simulink model "MPC_KIN_IPOPT_fast_no_param"  (R2018b)
settings: Solver=ode4  StartTime=0.0  StopTime=inf  FixedStep=Tsample  RelTol=1e-3
values from neighbouring files (symbols this model uses):
  N = evalin('base', 'N')    [solver_NLP_no_param.m]
undefined symbols (not defined in the file or in its folder): DiscIntNeverNeededParam, T, Tsample, x0_val, xd
libraries: simulink x2, templibrary x1
settings Model: Creator=francesco  LastModifiedBy=francesco
settings ModelReferenceCC: PropagateVarSize=Only when enabling

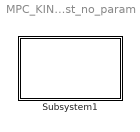
== system MPC_KIN_IPOPT_fast_no_param ==
  Subsystem1 : Subsystem  InitFcn=initialization_no_param

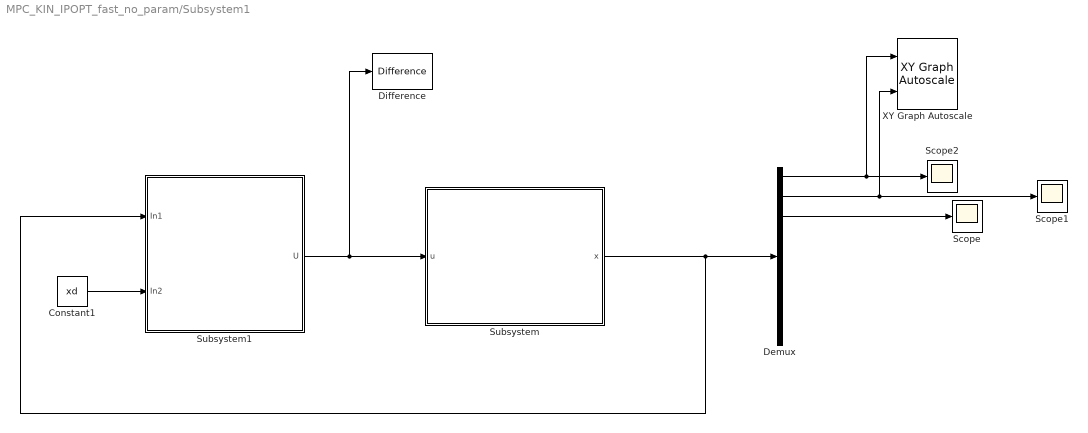
== system MPC_KIN_IPOPT_fast_no_param/Subsystem1 ==
  Constant1 : Constant  Value=xd
  Demux : Demux  Outputs=9
  Difference : simulink/Discrete/Difference  ICPrevInput=0.0  OutMin=[]  OutMax=[]  OutDataType=fixdt(1, 16)  OutScaling=2^-10  DoSatur=off
  Scope : Scope
  Scope1 : Scope
  Scope2 : Scope
  Subsystem : Subsystem
      mask Display: disp('{\bf\fontsize{10}KINEMATIC SYSTEM}', 'texmode','on');
  Subsystem1 : Subsystem
  XY Graph Autoscale : templibrary/XY Graph  Autoscale  xmin=-1  xmax=1  ymin=-1  ymax=1  st=-1
  wires:
  Subsystem/1(x) -> Demux/1, Subsystem1/1(In1)
  Demux/1 -> XY Graph Autoscale/1, Scope2/1
  Demux/3 -> Scope/1
  Demux/2 -> XY Graph Autoscale/2, Scope1/1
  Subsystem1/1(U) -> Difference/1, Subsystem/1(u)
  Constant1/1 -> Subsystem1/2(In2)

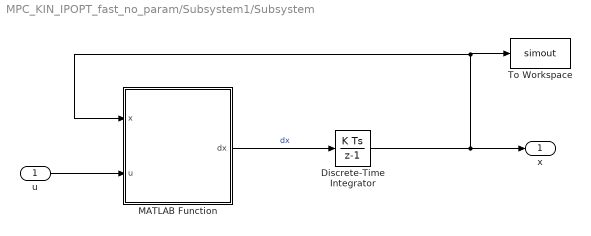
== system MPC_KIN_IPOPT_fast_no_param/Subsystem1/Subsystem ==
  u : Inport
  Discrete-Time Integrator : DiscreteIntegrator  InitialCondition=x0_val  SampleTime=Tsample  ICPrevOutput=DiscIntNeverNeededParam  ICPrevScaledInput=DiscIntNeverNeededParam
  MATLAB Function : MATLAB Function  TreatAsAtomicUnit=on
  To Workspace : ToWorkspace  VariableName=simout  SampleTime=T
  x : Outport  SampleTime=Tsample
  wires:
  u/1 -> MATLAB Function/2(u)
  MATLAB Function/1(dx) -> Discrete-Time Integrator/1  "dx"
  Discrete-Time Integrator/1 -> MATLAB Function/1(x), To Workspace/1, x/1

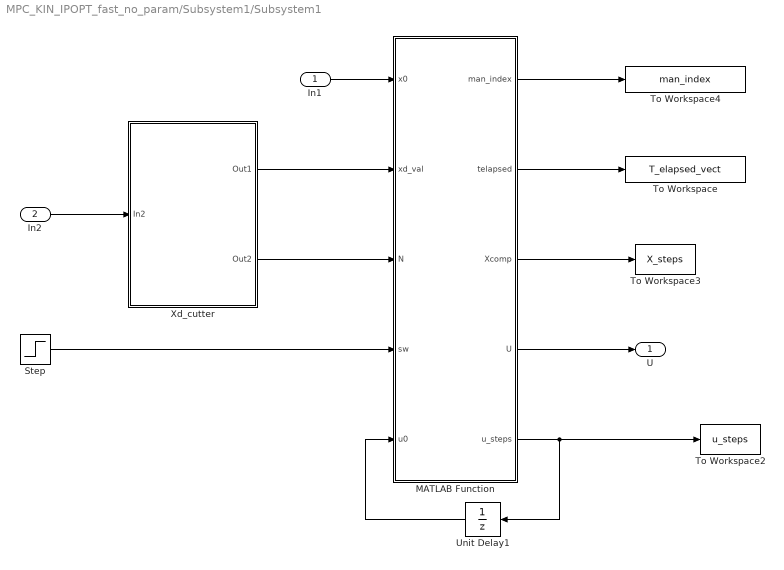
== system MPC_KIN_IPOPT_fast_no_param/Subsystem1/Subsystem1 ==
  In1 : Inport
  In2 : Inport  Port=2
  MATLAB Function : MATLAB Function  TreatAsAtomicUnit=on
  Step : Step  Time=0  SampleTime=0
  To Workspace : ToWorkspace  VariableName=T_elapsed_vect  SampleTime=T
  To Workspace2 : ToWorkspace  VariableName=u_steps  SaveFormat=Structure  SampleTime=-1
  To Workspace3 : ToWorkspace  VariableName=X_steps  SaveFormat=Structure  SampleTime=-1
  To Workspace4 : ToWorkspace  VariableName=man_index  SampleTime=T
  Unit Delay1 : UnitDelay  InitialCondition=zeros(8*N,1)  SampleTime=T
  Xd_cutter : Subsystem
  U : Outport
  wires:
  In1/1 -> MATLAB Function/1(x0)
  MATLAB Function/4(U) -> U/1
  MATLAB Function/2(telapsed) -> To Workspace/1
  Unit Delay1/1 -> MATLAB Function/5(u0)
  MATLAB Function/5(u_steps) -> Unit Delay1/1, To Workspace2/1
  MATLAB Function/3(Xcomp) -> To Workspace3/1
  In2/1 -> Xd_cutter/1(In2)
  Xd_cutter/1(Out1) -> MATLAB Function/2(xd_val)
  Xd_cutter/2(Out2) -> MATLAB Function/3(N)
  Step/1 -> MATLAB Function/4(sw)
  MATLAB Function/1(man_index) -> To Workspace4/1

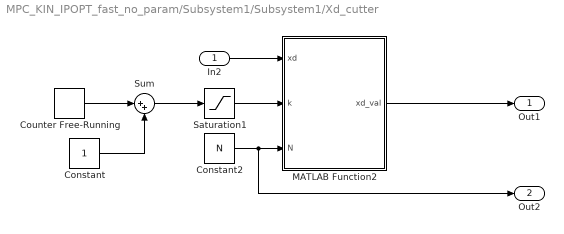
== system MPC_KIN_IPOPT_fast_no_param/Subsystem1/Subsystem1/Xd_cutter ==
  In2 : Inport
  Constant : Constant
  Constant2 : Constant  Value=N
  Counter Free-Running : simulink/Sources/Counter Free-Running  NumBits=12  tsamp=T
  MATLAB Function2 : MATLAB Function  TreatAsAtomicUnit=on
  Saturation1 : Saturate  UpperLimit=size(xd,2)
  Sum : Sum  Inputs=|++
  Out1 : Outport
  Out2 : Outport  Port=2
  wires:
  Counter Free-Running/1 -> Sum/1
  Saturation1/1 -> MATLAB Function2/2(k)
  MATLAB Function2/1(xd_val) -> Out1/1
  Sum/1 -> Saturation1/1
  Constant/1 -> Sum/2
  Constant2/1 -> Out2/1, MATLAB Function2/3(N)
  In2/1 -> MATLAB Function2/1(xd)

== matlab function MPC_KIN_IPOPT_fast_no_param/Subsystem1/Subsystem1/MATLAB Function ==
  settings: updateMethod=DISCRETE  sampleTime=T
  data: man_index output size=[1]; telapsed output; Xcomp output size=[15,N+1]; U output; u_steps output double size=[8*N,1]; x0 input; xd_val input; N input; sw input; u0 input
function [man_index,telapsed,Xcomp,U,u_steps] = fnc(x0,xd_val,N,sw,u0)

coder.extrinsic('solver_NLP_no_param');


u_steps=zeros(8*25,1);
% INITIALIZING VARIABLES

telapsed=0;
unew=zeros(8*N,1);
U=zeros(8,1);
Xcomp=zeros(15,N);
man_index=0;

% SOLVING THE PROBLEM

[ U, unew, Xcomp, telapsed, man] = solver_NLP_no_param(xd_val,x0,u0,sw);

man_index(1)=man;
u_steps=unew(1:8*25,1);

end

== matlab function MPC_KIN_IPOPT_fast_no_param/Subsystem1/Subsystem1/Xd_cutter/MATLAB Function2 ==
  settings: updateMethod=DISCRETE  sampleTime=T
  data: xd input; k input; N input; xd_val output size=[15,N]
function xd_val = fcn(xd,k,N)

xd_val=zeros(15,N);

if size(xd,2)-k>N-1
h=xd(:,k+1:k+N);
      
else
h=[xd(:,k+1:end) xd(:,end)*ones(1,N-(size(xd,2)-k))];

end
xd_val = h;

end

== matlab function MPC_KIN_IPOPT_fast_no_param/Subsystem1/Subsystem/MATLAB Function ==
  settings: updateMethod=DISCRETE  sampleTime=Tsample
  data: x input; dx output; u input size=[8 1]
function dx = sys_dynamics(x,u)


G=[cos(x(3)) 0; sin(x(3)) 0; 0 1 ];

B = zeros(6,2);

dx = [   G                zeros(3,6)  ; ...
         zeros(6,2)       eye(6)      ; ...
         zeros(6,8)                   ]*u;

end
